simulink model "FOC_2020b"  (R2021a)
settings: Solver=ode23t  StartTime=0.0  StopTime=0.1  RelTol=1e-3  AbsTol=1e-3  EnableMultiTasking=on
values from neighbouring files (symbols this model uses):
  f_c = 10000    [FOC_params.m]
  Kpd = Ld*2*pi*BW    (= 0.0753982236862)    [FOC_params.m]
  Kpn = Kpq/(Lq*d*K)    (= 1.22461076833)    [FOC_params.m]
  Kpq = Lq*2*pi*BW    (= 0.125663706144)    [FOC_params.m]
  Kr = 270    [FOC_params.m]
  Ld = 0.00003    (= 3e-05)    [FOC_params.m]
  Lq = 0.00005    (= 5e-05)    [FOC_params.m]
  np = 5    [FOC_params.m]
  PERIOD = 3750    [FOC_params.m]
  psiPM = 0.007    [FOC_params.m]
  R = 0.023    [FOC_params.m]
  T_dead = 2.0e-6    (= 2e-06)    [FOC_params.m]
  Tnd = Ld/R    (= 0.00130434782609)    [FOC_params.m]
  Tnn = d^2*Lq/Kpq    (= 0.039788735773)    [FOC_params.m]
  Tnq = Lq/R    (= 0.00217391304348)    [FOC_params.m]
  u_dc = 12    [FOC_params.m]
libraries: nesl_utility x23, ee_lib x22, fl_lib x22, pid_lib x3, simulink x3, cstblocks x2, spsAlphaBetaZerotodq0Lib x1, spsabctoAlphaBetaZeroLib x1, spsdq0toAlphaBetaZeroLib x1, spsTriangleGeneratorLib x1
(part 1 of 2)
settings Model: Creator=Michael Hoerner  LastModifiedBy=wilflingti
settings SolverCC: AutoScaleAbsTol=off  AlgebraicLoopSolver=TrustRegion  DecoupledContinuousIntegration=on  MinimalZcImpactIntegration=on
settings DataIOCC: LimitDataPoints=on  MaxDataPoints=10000  ReturnWorkspaceOutputs=off
settings OptimizationCC: StrengthReduction=on  PassReuseOutputArgsAs=Individual arguments  OptimizeBlockOrder=speed  OptimizationPriority=Speed  OptimizationCustomize=off  MultiThreadedLoops=on  EfficientTunableParamExpr=on
settings DebuggingCC: ParameterTunabilityLossMsg=error  AllowSymbolicDim=off  SFUnexpectedBacktrackingDiag=warning  SFNoUnconditionalDefaultTransitionDiag=warning  SFExecutionAtInitializationDiag=none  SFMachineParentedDataDiag=warning  ArithmeticOperatorsInVariantConditions=warning
settings HardwareCC: ProdBitPerChar=16  ProdBitPerInt=16  ProdBitPerPointer=32  ProdBitPerSizeT=32  ProdBitPerPtrDiffT=32  ProdLargestAtomicInteger=Integer  ProdLargestAtomicFloat=None  ProdWordSize=16  ProdHWDeviceType=Texas Instruments->C2000
settings SFSimCC: SimUseLocalCustomCode=off  MATLABDynamicMemAlloc=off  CustomCodeUndefinedFunction=UseInterfaceOnly
settings RTWCC: SystemTargetFile=ert.tlc  TemplateMakefile=ert_default_tmf  GenerateReport=on  RTWUseLocalCustomCode=off  IncludeHyperlinkInReport=on  LaunchReport=on  GenerateTraceInfo=on  GenerateTraceReport=on  GenerateTraceReportSl=on  GenerateTraceReportSf=on  GenerateTraceReportEml=on
settings CodeAppCC: ForceParamTrailComments=on  IgnoreCustomStorageClasses=off  OperatorAnnotations=on  SimulinkDataObjDesc=on  SFDataObjDesc=on  InsertBlockDesc=on
settings ERTTargetCC: CodeReplacementLibrary=TI C28x with C99 extensions  GenerateSampleERTMain=on  CodeInterfacePackaging=Reusable function  MultiInstanceErrorCode=Warning  ERTCustomFileTemplate=example_file_process.tlc  ERTFilePackagingFormat=Compact
settings ConfigComp: CovMetricSettings=dw  CovSaveCumulativeToWorkspaceVar=on  CovSaveSingleToWorkspaceVar=on  CovExternalEMLEnable=off  CovSFcnEnable=off
settings SimscapeCC: SimscapeLogDataHistory=10000

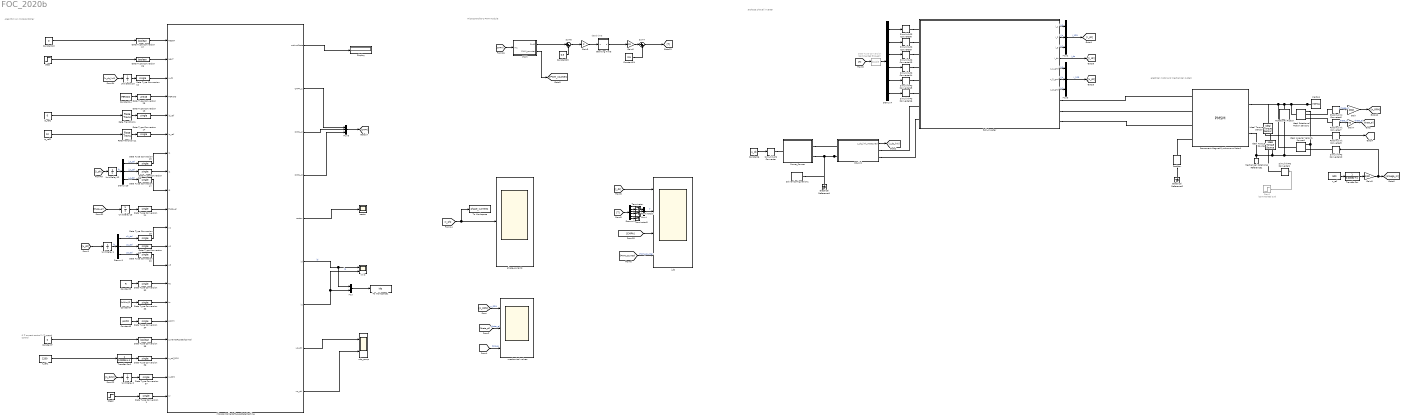
== system FOC_2020b ==
  note: electrical motor and mechanical system
  note: 3-phase 2-level inverter
  note: dead time
  note: Microcontroller's PWM module
  note: Algorithm on microcontroller
  note: 0 = current control
      | 1 = speed control
  3ph_Inverter : Subsystem
  Blanking Time : Subsystem  mask(Blanking Time){tb=T_dead}
      mask prompts: tb "Delay time:"
      mask help:
      | This block generates a blanking time for two-level inverter bridges so that the turn-on of one switch is delayed with respect to the turn-off of the other switch in the inverter leg.
      |
      | The input s is a switching function generated by a 2-level modulator. The values of the output s' are either 1, 0 or -1. If the input is a vector, the output is also a vector of the same width.
      mask Help: eval('plecs(''help'', ''blankingtime.html'')')
  Constant10 : Constant  Value=0
  Constant14 : Constant  Value=PERIOD
  Constant23 : Constant  Value=0.5
  Constant24 : Constant  Value=0.5
  Constant3 : Constant  Value=R
  Constant4 : Constant  Value=(Ld+Lq)/2
  Constant5 : Constant  Value=psiPM
  Constant6 : Constant  Value=u_dc
  Constant7 : Constant  Value=0
  DC_link : Subsystem
  Data Type Conversion : DataTypeConversion  Commented=through  OutDataTypeStr=double
  Data Type Conversion{1,12..21,32..34,36..37} (16 alike) : DataTypeConversion  OutDataTypeStr=single
  Data Type Conversion25 : DataTypeConversion  OutDataTypeStr=uint16
  Data Type Conversion26 : DataTypeConversion  OutDataTypeStr=boolean
  Data Type Conversion27 : DataTypeConversion  OutDataTypeStr=boolean
  Data Type Conversion35 : DataTypeConversion  OutDataTypeStr=boolean
  Demux1 : Demux  Outputs=3
  Demux10 : Demux  Outputs=3
  Demux3 : Demux  Outputs=6
  Demux4 : Demux  Outputs=6
  Display : Display
  Electrical Reference1 : fl_lib/Electrical/Electrical Elements/Electrical Reference
  Electrical Reference2 : fl_lib/Electrical/Electrical Elements/Electrical Reference
  Gain : Gain  Gain=30/pi
  Gain5 : Gain  Gain=2
  Gain6 : Gain  Gain=0.5
  Gain7 : Gain  Gain=np
  Gain8 : Gain  Gain=pi/30
  Ideal Angular Velocity Source1 : fl_lib/Mechanical/Mechanical Sources/Ideal Angular Velocity Source
  Ideal Rotational Motion Sensor1 : fl_lib/Mechanical/Mechanical Sensors/Ideal Rotational Motion Sensor  wrap_angle=simscape.enum.onoff.off  offset=0 deg
  Ideal Torque Sensor : fl_lib/Mechanical/Mechanical Sensors/Ideal Torque Sensor
  Ideal Torque Source : fl_lib/Mechanical/Mechanical Sources/Ideal Torque Source
  Inertia1 : fl_lib/Mechanical/Rotational Elements/Inertia  inertia=J kg*m^2  num_ports=foundation.enum.numPorts2.one  w_specify=off  w_priority=High  w=0 rad/s  w_nominal_specify=off  w_nominal_unit=rad/s  w_nominal_value=1  t_specify=off  t_priority=None  t=0 N*m  t_nominal_specify=off  t_nominal_unit=N*m  t_nominal_value=1
  Mechanical Rotational Reference1 : fl_lib/Mechanical/Rotational Elements/Mechanical Rotational Reference
  MicrocontrollerSoftwareStateMachine : Stateflow chart  TreatAsAtomicUnit=on
  Mux : Mux  Inputs=2
  Mux{2..4,6} (4 alike) : Mux  Inputs=3
  PS-Simulink Converter6 : nesl_utility/PS-Simulink Converter  PhysicalDomain=network_engine_domain  SubClassName=ps_output  LeftPortType=input  RightPortType=output  PseudoPeriodic=off  Frequencies=[]  Unit=1  AffineConversion=off
      settings: SourceProductBaseCode=PW,SS
  PS-Simulink Converter7 : nesl_utility/PS-Simulink Converter  PhysicalDomain=network_engine_domain  SubClassName=ps_output  LeftPortType=input  RightPortType=output  PseudoPeriodic=off  Frequencies=[]  Unit=1  AffineConversion=off
      settings: SourceProductBaseCode=PW,SS
  PS-Simulink Converter8 : nesl_utility/PS-Simulink Converter  PhysicalDomain=network_engine_domain  SubClassName=ps_output  LeftPortType=input  RightPortType=output  PseudoPeriodic=off  Frequencies=[]  Unit=1  AffineConversion=off
      settings: SourceProductBaseCode=PW,SS
  PWM : Subsystem
  Permanent Magnet Synchronous Motor1 : ee_lib/Electromechanical/Permanent Magnet/PMSM  winding_type=ee.enum.statorconnection.wye  machine_param=ee.enum.pmsm.parameterization.constant  nPolePairs=np  pmflux_param=1  pm_flux_linkage=psiPM Wb  torque_constant=0.18 N*m/A  back_emf_constant=0.18 V/(rad/s)  stator_param=1  Ld=Ld H  Lq=Lq H  idVec=[-200, 0, 200] A  iqVec=[-200, 0, 200] A  LdMatrix=0.0002 * ones(3, 3) H  LqMatrix=0.0002 * ones(3, 3) H  PmMatrix=0.1 * ones(3, 3) Wb  ktMatrix=0.18 * ones(3, 3) N*m/A  keMatrix=0.18 * ones(3, 3) V/(rad/s)  L0=0.00016 H  Ls=0.0002 H  Lm=-0.00002 H  Ms=0.00002 H  Rs=R Ohm  zero_sequence=ee.enum.park.zerosequence.include  J=0.0 kg*m^2  lam=0 N*m/(rad/s)  axes_param=2  i_d_specify=off  i_d_priority=None  i_d=0 A  i_d_nominal_specify=off  i_d_nominal_unit=A  i_d_nominal_value=1  i_q_specify=off  i_q_priority=None  i_q=0 A  i_q_nominal_specify=off  i_q_nominal_unit=A  i_q_nominal_value=1  torque_specify=off  torque_priority=None  torque=0 N*m  torque_nominal_specify=off  torque_nominal_unit=N*m  torque_nominal_value=1  angular_velocity_specify=off  angular_velocity_priority=High  angular_velocity=0 deg/s  angular_velocity_nominal_specify=off  angular_velocity_nominal_unit=rpm  angular_velocity_nominal_value=1  angular_position_specify=off  angular_position_priority=High  angular_position=0 deg  angular_position_nominal_specify=off  angular_position_nominal_unit=deg  angular_position_nominal_value=1  loss_param=ee.enum.ironloss.none  losses_oc=[0, 0, 0] W  losses_sc=[0, 0, 0] W  f_losses=60 Hz  Isc_losses=95 A  Tmeas=298.15 K  alpha=3.93e-3 1/K  alpha_flux=-0.001 1/K  stator_thermal_mass=100 J/K  rotor_thermal_mass=200 J/K  Rm_percent_rotor=90  Rd_percent_rotor=30  temperatureA_specify=off  temperatureA_priority=High  temperatureA=25 degC  temperatureA_nominal_specify=off  temperatureA_nominal_unit=degC  temperatureA_nominal_value=1  temperatureB_specify=off  temperatureB_priority=High  temperatureB=25 degC  temperatureB_nominal_specify=off  temperatureB_nominal_unit=degC  temperatureB_nominal_value=1  temperatureC_specify=off  temperatureC_priority=High  temperatureC=25 degC  temperatureC_nominal_specify=off  temperatureC_nominal_unit=degC  temperatureC_nominal_value=1  temperatureR_specify=off  temperatureR_priority=High  temperatureR=25 degC  temperatureR_nominal_specify=off  temperatureR_nominal_unit=degC  temperatureR_nominal_value=1
      settings: InternalSimscapePortConfiguration="{\"Bottom\":[],\"Left\":[{\"id\":\"a\",\"label\":\"a\",\"type\":\"foundation.electrical.electrical\"},{\"id\":\"b\",\"label\":\"b\",\"type\":\"foundation.electrical.electrical\"},{\"id\":\"c\",\"label\":\"c\",\"type\":\"foundation.electrical.electrical\"},{\"id\":\"n\",\"label\":\"n\",\"type\":\"foundation.electrical.electrical\"}],\"Right\":[{\"id\":\"R\",\"label\":\"R\",\"type\":\"foundation.mechanical.rotational.rotational\"},{\"id\":\"C\",\"label\":\"C\",\"type\":\"foundation.mechanical.rotational.rotational\"}],\"Top\":[]}"
  Power_Source : Subsystem
  Rate Transition1 : RateTransition  OutPortSampleTime=1/f_c
  Rate Transition11 : RateTransition  OutPortSampleTime=1/f_c
  Resistor : fl_lib/Electrical/Electrical Elements/Resistor  R=2e6 Ohm  i_specify=off  i_priority=None  i=0 A  i_nominal_specify=off  i_nominal_unit=A  i_nominal_value=1  v_specify=off  v_priority=None  v=0 V  v_nominal_specify=off  v_nominal_unit=V  v_nominal_value=1
  Rotational Friction : fl_lib/Mechanical/Rotational Elements/Rotational Friction  brkwy_trq=0.0622476 N*m  brkwy_vel=0.1 rad/s  Col_trq=0.03460117 N*m  visc_coef=0.00026373 N*m/(rad/s)  w_specify=off  w_priority=None  w=0 rad/s  w_nominal_specify=off  w_nominal_unit=rad/s  w_nominal_value=1  t_specify=off  t_priority=None  t=0 N*m  t_nominal_specify=off  t_nominal_unit=N*m  t_nominal_value=1
  Simulink-PS Converter{,8..9,13..16} (7 alike) : nesl_utility/Simulink-PS Converter  PhysicalDomain=network_engine_domain  SubClassName=ps_input  LeftPortType=input  RightPortType=output  PseudoPeriodic=off  Frequencies=[]  NoiseDistribution=none  NoiseParameters=[]  Unit=1  AffineConversion=off  FilteringAndDerivatives=provide  SimscapeFilterOrder=1  InputFilterTimeConstant=0.001  UdotUserProvided=0
      settings: SourceProductBaseCode=PW,SS
  Simulink-PS Converter1 : nesl_utility/Simulink-PS Converter  PhysicalDomain=network_engine_domain  SubClassName=ps_input  LeftPortType=input  RightPortType=output  PseudoPeriodic=off  Frequencies=[]  NoiseDistribution=none  NoiseParameters=[]  Unit=1  AffineConversion=off  FilteringAndDerivatives=filter  SimscapeFilterOrder=1  InputFilterTimeConstant=0.001  UdotUserProvided=0
      settings: SourceProductBaseCode=PW,SS
  Simulink-PS Converter10 : nesl_utility/Simulink-PS Converter  PhysicalDomain=network_engine_domain  SubClassName=ps_input  LeftPortType=input  RightPortType=output  PseudoPeriodic=off  Frequencies=[]  NoiseDistribution=none  NoiseParameters=[]  Unit=1  AffineConversion=off  FilteringAndDerivatives=filter  SimscapeFilterOrder=1  InputFilterTimeConstant=0.001  UdotUserProvided=0
      settings: SourceProductBaseCode=PW,SS
  Solver Configuration1 : nesl_utility/Solver Configuration  PhysicalDomain=network_engine_domain  SubClassName=solver  LeftPortType=input  RightPortType=generic  Tones=[]  Harmonics=[]  SimulateNoise=off  Profile=off  UseLocalSampling=off  EnableSwitchedLinearOptims=on  FrequencyDomain=off  UseCCode=off  RelTol=0.001  AbsTol=1e-06  MinStep=1e-09  ToWorkspace=off  RevertToSquareIcSolve=off  NumHomotopyIterations=100  PhasorMode=off  PhasorModeNumHarmonics=1  DoDC=off  ResidualTolerance=1e-09  UseLocalSolver=off  LocalSolverChoice=NE_BACKWARD_EULER_ADVANCER  LocalSolverSampleTime=1e-6  DoFixedCost=off  MaxNonlinIter=3  MaxModeIter=2  ComputeImpulses=off  ImpulseIterations=2  LinearAlgebra=Sparse  EquationFormulation=NE_TIME_EF  DelaysMemoryBudget=1024  AutomaticFiltering=on  FilteringTimeConstant=0.001  PartitionStorageMethod=AS_NEEDED  PartitionMemoryBudget=1024  PartitionMethod=FAST
      settings: SourceProductBaseCode=PW,SS
  Step : Step  Time=2/f_c  Before=1  After=0  SampleTime=0
  Step1 : Step  Commented=on  Time=0.08  After=-0.5  SampleTime=0
  Step2 : Step  Time=0.04  After=Kr  SampleTime=0
  Sum6 : Sum  Inputs=|+-
  Sum7 : Sum  Inputs=|++
  Terminator : Terminator
  Terminator1 : Terminator
  Terminator3 : Terminator
  To Workspace : ToWorkspace  VariableName=phase_currents  SaveFormat=Timeseries  SampleTime=1/1000
  To Workspace1 : ToWorkspace  VariableName=idq  SaveFormat=Timeseries  SampleTime=1/1000
  Transfer Fcn : TransferFcn  Denominator=[0.0005 1]
  Transfer Fcn1 : TransferFcn  Denominator=[0.0005 1]
  Unit Delay{1..2,10,12..13} (5 alike) : UnitDelay  SampleTime=1/f_c  HasFrameUpgradeWarning=on
  i_dc : Scope  NumInputPorts=4
  id,iq : Scope  NumInputPorts=2
  id_ref2 : Constant  Value=0
  iq_ref2 : Constant  Value=10
  mechanical values : Scope  NumInputPorts=3
  n_ref : Constant  Value=500
  n_ref1 : Constant  Value=1200
  phase_currents : Scope
  "sector " : Scope
  udq_comp : Scope  NumInputPorts=2
  wires:
  DC_link/1(u_dc_link_measured) -> [u_dc_link]
  Constant6/1 -> Simulink-PS Converter/1
  3ph_Inverter/3(i_3) -> Mux2/3  "i_c"
  3ph_Inverter/2(i_2) -> Mux2/2  "i_b"
  Mux2/1 -> [i_ph]  "i_123"
  PS-Simulink Converter7/1 -> Gain7/1  "theta_m"
  Gain7/1 -> [theta_el]  "theta_el"
  Gain8/1 -> Simulink-PS Converter10/1, [omega_m]
  PS-Simulink Converter6/1 -> Gain/1  "omega_m"
  PS-Simulink Converter8/1 -> [torque]
  [T] -> Demux3/1
  Demux3/1 -> Mux4/1
  Demux3/3 -> Mux4/2
  Demux3/5 -> Mux4/3
  Demux3/2 -> Terminator/1
  Demux3/4 -> Terminator1/1
  [PWM_counter] -> i_dc/4  "PWM_counter"
  3ph_Inverter/1(i_1) -> Mux2/1  "i_a"
  3ph_Inverter/4(i_dc) -> [i_dc]  "i_dc"
  [i_dc] -> i_dc/1
  Demux3/6 -> Terminator3/1
  [T] -> Data Type Conversion/1
  [i_ph] -> To Workspace/1, phase_currents/1
  Mux4/1 -> i_dc/2  "T"
  n_ref/1 -> Transfer Fcn/1
  Data Type Conversion12/1 -> MicrocontrollerSoftwareStateMachine/3(u_dc)
  Data Type Conversion13/1 -> MicrocontrollerSoftwareStateMachine/5(id_ref)
  Data Type Conversion14/1 -> MicrocontrollerSoftwareStateMachine/6(iq_ref)
  Data Type Conversion15/1 -> MicrocontrollerSoftwareStateMachine/7(i1)
  Data Type Conversion16/1 -> MicrocontrollerSoftwareStateMachine/8(i2)
  Data Type Conversion17/1 -> MicrocontrollerSoftwareStateMachine/9(i3)
  Data Type Conversion21/1 -> MicrocontrollerSoftwareStateMachine/10(theta_el)
  Data Type Conversion25/1 -> MicrocontrollerSoftwareStateMachine/4(PERIOD)
  Data Type Conversion26/1 -> MicrocontrollerSoftwareStateMachine/2(NEXT)
  Data Type Conversion27/1 -> MicrocontrollerSoftwareStateMachine/1(RESET)
  Constant10/1 -> Data Type Conversion27/1
  Step/1 -> Data Type Conversion26/1
  Unit Delay10/1 -> Data Type Conversion12/1
  [u_dc_link] -> Unit Delay10/1
  Constant14/1 -> Data Type Conversion25/1
  Rate Transition11/1 -> Data Type Conversion14/1
  id_ref2/1 -> Rate Transition1/1
  iq_ref2/1 -> Rate Transition11/1
  Rate Transition1/1 -> Data Type Conversion13/1
  Demux10/3 -> Data Type Conversion17/1  "i_c_ctrl"
  Unit Delay12/1 -> Demux10/1  "fc"
  Demux10/1 -> Data Type Conversion15/1  "i_a_ctrl"
  Demux10/2 -> Data Type Conversion16/1  "i_b_ctrl"
  [i_ph] -> Unit Delay12/1
  [theta_el] -> Unit Delay13/1
  Unit Delay13/1 -> Data Type Conversion21/1
  MicrocontrollerSoftwareStateMachine/3(CMPA_2) -> Mux6/2
  MicrocontrollerSoftwareStateMachine/2(CMPA_1) -> Mux6/1
  MicrocontrollerSoftwareStateMachine/4(CMPA_3) -> Mux6/3
  MicrocontrollerSoftwareStateMachine/5(sector) -> "sector "/1
  Transfer Fcn/1 -> Gain8/1
  [CMPA] -> i_dc/3
  Mux6/1 -> [CMPA]
  Demux1/2 -> Data Type Conversion19/1  "u2_ctrl"
  Unit Delay1/1 -> Demux1/1  "fc"
  Demux1/1 -> Data Type Conversion18/1  "u1_ctrl"
  [u_ph] -> Unit Delay1/1
  Demux1/3 -> Data Type Conversion20/1  "u3_ctrl"
  Data Type Conversion19/1 -> MicrocontrollerSoftwareStateMachine/12(u2)
  Data Type Conversion18/1 -> MicrocontrollerSoftwareStateMachine/11(u1)
  Data Type Conversion20/1 -> MicrocontrollerSoftwareStateMachine/13(u3)
  Data Type Conversion32/1 -> MicrocontrollerSoftwareStateMachine/14(Rs)
  Data Type Conversion33/1 -> MicrocontrollerSoftwareStateMachine/15(Ls)
  Data Type Conversion34/1 -> MicrocontrollerSoftwareStateMachine/16(psiPM)
  Constant3/1 -> Data Type Conversion32/1
  Constant4/1 -> Data Type Conversion33/1
  Constant5/1 -> Data Type Conversion34/1
  3ph_Inverter/5(u_1_gnd) -> Mux3/1  "i_a"
  Mux3/1 -> [u_ph]  "i_123"
  3ph_Inverter/6(u_2_gnd) -> Mux3/2  "i_b"
  3ph_Inverter/7(u_3_gnd) -> Mux3/3  "i_c"
  Data Type Conversion35/1 -> MicrocontrollerSoftwareStateMachine/17(currentORspeedControl)
  Data Type Conversion36/1 -> MicrocontrollerSoftwareStateMachine/18(n_ref_RPM)
  Data Type Conversion37/1 -> MicrocontrollerSoftwareStateMachine/19(n_RPM)
  Constant7/1 -> Data Type Conversion35/1
  Gain/1 -> [n_RPM]
  Unit Delay2/1 -> Data Type Conversion37/1
  [n_RPM] -> Unit Delay2/1
  Transfer Fcn1/1 -> Data Type Conversion36/1
  Step1/1 -> Simulink-PS Converter1/1
  MicrocontrollerSoftwareStateMachine/6(id) -> Mux/1, id,iq/1  "id"
  MicrocontrollerSoftwareStateMachine/7(iq) -> Mux/2, id,iq/2  "iq"
  Data Type Conversion/1 -> Demux4/1
  PWM/2(PWM_counter) -> [PWM_counter]
  Demux4/1 -> Simulink-PS Converter8/1
  Demux4/2 -> Simulink-PS Converter9/1
  Demux4/3 -> Simulink-PS Converter13/1
  Demux4/4 -> Simulink-PS Converter14/1
  Demux4/5 -> Simulink-PS Converter15/1
  Demux4/6 -> Simulink-PS Converter16/1
  Gain5/1 -> Blanking Time/1(s)
  Constant23/1 -> Sum6/2
  Gain6/1 -> Sum7/1
  Blanking Time/1(s') -> Gain6/1
  Constant24/1 -> Sum7/2
  Sum6/1 -> Gain5/1
  Sum7/1 -> [T]
  PWM/1(Out1) -> Sum6/1
  MicrocontrollerSoftwareStateMachine/8(ud_ctrl) -> udq_comp/1
  MicrocontrollerSoftwareStateMachine/9(uq_ctrl) -> udq_comp/2
  n_ref1/1 -> Transfer Fcn1/1
  [CMPA] -> PWM/1(In1)
  MicrocontrollerSoftwareStateMachine/1(activeState) -> Display/1
  [torque] -> mechanical values/3  "torque"
  [n_RPM] -> mechanical values/1  "n_RPM"
  [theta_el] -> mechanical values/2  "theta_el"
  Data Type Conversion1/1 -> MicrocontrollerSoftwareStateMachine/20(Kr)
  Step2/1 -> Data Type Conversion1/1
  Mux/1 -> To Workspace1/1
  connections:
  DC_link/LConn2 -- Power_Source/RConn2 -- Solver Configuration1/RConn1 -- Electrical Reference1/LConn1
  Inertia1/LConn1 -- Ideal Angular Velocity Source1/LConn1 -- Permanent Magnet Synchronous Motor1/RConn1 -- Ideal Torque Sensor/LConn1 -- Rotational Friction/LConn1 -- Ideal Rotational Motion Sensor1/LConn1
  Ideal Rotational Motion Sensor1/RConn1 -- Ideal Angular Velocity Source1/RConn2 -- Rotational Friction/RConn1 -- Permanent Magnet Synchronous Motor1/RConn2 -- Mechanical Rotational Reference1/LConn1 -- Ideal Torque Source/RConn2
  Simulink-PS Converter14/RConn1 -- 3ph_Inverter/LConn4
  Simulink-PS Converter15/RConn1 -- 3ph_Inverter/LConn5
  Simulink-PS Converter16/RConn1 -- 3ph_Inverter/LConn6
  Power_Source/RConn1 -- DC_link/LConn1
  PS-Simulink Converter6/LConn1 -- Ideal Rotational Motion Sensor1/RConn2
  Simulink-PS Converter/RConn1 -- Power_Source/LConn1
  Simulink-PS Converter8/RConn1 -- 3ph_Inverter/LConn1
  Simulink-PS Converter9/RConn1 -- 3ph_Inverter/LConn2
  DC_link/RConn1 -- 3ph_Inverter/LConn7
  Simulink-PS Converter13/RConn1 -- 3ph_Inverter/LConn3
  DC_link/RConn2 -- 3ph_Inverter/LConn8
  PS-Simulink Converter7/LConn1 -- Ideal Rotational Motion Sensor1/RConn3
  3ph_Inverter/RConn1 -- Permanent Magnet Synchronous Motor1/LConn1
  3ph_Inverter/RConn2 -- Permanent Magnet Synchronous Motor1/LConn2
  3ph_Inverter/RConn3 -- Permanent Magnet Synchronous Motor1/LConn3
  Resistor/LConn1 -- Permanent Magnet Synchronous Motor1/LConn4
  Simulink-PS Converter10/RConn1 -- Ideal Angular Velocity Source1/RConn1
  PS-Simulink Converter8/LConn1 -- Ideal Torque Sensor/RConn2
  Resistor/RConn1 -- Electrical Reference2/LConn1
  Simulink-PS Converter1/RConn1 -- Ideal Torque Source/RConn1
  Ideal Torque Source/LConn1 -- Ideal Torque Sensor/RConn1

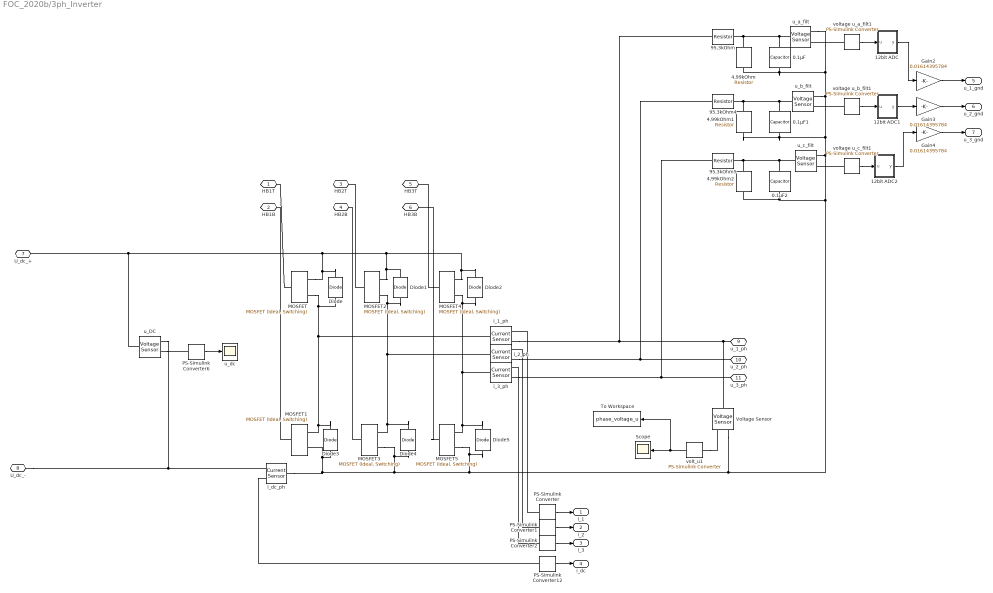
== system FOC_2020b/3ph_Inverter ==
  0.1µF : ee_lib/Passive/Capacitor  cap_option=0  c=0.1 uF  Cvec=[ 1e-5 1e-6 ] F  Vvec=[ 0 10 ] V  CV_table_symmetry=1  f_vec=[1, 10] kHz  DFext_vec=[.8, 1.2]  C_tol=5  enable_C_tol=0  tol_distribution=1  nSigma=4  r=1e-6 Ohm  g=0 1/Ohm  averaging_period=0 s  enable_operating_limits=0  operating_limit_action=2  max_working_voltage_range=[ -25 25 ] V  power_rating=1 W  enable_faults=0  fault_action=1  Cscale_faulted=100  R_faulted=0.001 Ohm  G_faulted=0 1/Ohm  tau_fault=0.001 s  enable_temporal_fault=0  t_fault=1 s  enable_behavioral_fault=0  max_permissible_voltage_range=[ -100 100 ] V  t_fail_on_voltage=1 s  i_specify=off  i_priority=None  i=0 A  i_nominal_specify=off  i_nominal_unit=A  i_nominal_value=1  v_specify=off  v_priority=None  v=0 V  v_nominal_specify=off  v_nominal_unit=V  v_nominal_value=1  vc_specify=on  vc_priority=High  vc=0 V  vc_nominal_specify=off  vc_nominal_unit=V  vc_nominal_value=1
  0.1µF1 : ee_lib/Passive/Capacitor  cap_option=0  c=0.1 uF  Cvec=[ 1e-5 1e-6 ] F  Vvec=[ 0 10 ] V  CV_table_symmetry=1  f_vec=[1, 10] kHz  DFext_vec=[.8, 1.2]  C_tol=5  enable_C_tol=0  tol_distribution=1  nSigma=4  r=1e-6 Ohm  g=0 1/Ohm  averaging_period=0 s  enable_operating_limits=0  operating_limit_action=2  max_working_voltage_range=[ -25 25 ] V  power_rating=1 W  enable_faults=0  fault_action=1  Cscale_faulted=100  R_faulted=0.001 Ohm  G_faulted=0 1/Ohm  tau_fault=0.001 s  enable_temporal_fault=0  t_fault=1 s  enable_behavioral_fault=0  max_permissible_voltage_range=[ -100 100 ] V  t_fail_on_voltage=1 s  i_specify=off  i_priority=None  i=0 A  i_nominal_specify=off  i_nominal_unit=A  i_nominal_value=1  v_specify=off  v_priority=None  v=0 V  v_nominal_specify=off  v_nominal_unit=V  v_nominal_value=1  vc_specify=on  vc_priority=High  vc=0 V  vc_nominal_specify=off  vc_nominal_unit=V  vc_nominal_value=1
  0.1µF2 : ee_lib/Passive/Capacitor  cap_option=0  c=0.1 uF  Cvec=[ 1e-5 1e-6 ] F  Vvec=[ 0 10 ] V  CV_table_symmetry=1  f_vec=[1, 10] kHz  DFext_vec=[.8, 1.2]  C_tol=5  enable_C_tol=0  tol_distribution=1  nSigma=4  r=1e-6 Ohm  g=0 1/Ohm  averaging_period=0 s  enable_operating_limits=0  operating_limit_action=2  max_working_voltage_range=[ -25 25 ] V  power_rating=1 W  enable_faults=0  fault_action=1  Cscale_faulted=100  R_faulted=0.001 Ohm  G_faulted=0 1/Ohm  tau_fault=0.001 s  enable_temporal_fault=0  t_fault=1 s  enable_behavioral_fault=0  max_permissible_voltage_range=[ -100 100 ] V  t_fail_on_voltage=1 s  i_specify=off  i_priority=None  i=0 A  i_nominal_specify=off  i_nominal_unit=A  i_nominal_value=1  v_specify=off  v_priority=None  v=0 V  v_nominal_specify=off  v_nominal_unit=V  v_nominal_value=1  vc_specify=on  vc_priority=High  vc=0 V  vc_nominal_specify=off  vc_nominal_unit=V  vc_nominal_value=1
  12bit ADC : MATLAB Function  TreatAsAtomicUnit=on
  12bit ADC1 : MATLAB Function  TreatAsAtomicUnit=on
  12bit ADC2 : MATLAB Function  TreatAsAtomicUnit=on
  4,99kOhm : ee_lib/Passive/Resistor  R=4990 Ohm  R_tol=5  enable_R_tol=0  tol_distribution=1  nSigma=4  enable_operating_limits=0  operating_limit_action=2  max_working_voltage=100 V  power_rating=1 W  enable_faults=0  fault_action=1  R_faulted=Inf Ohm  enable_temporal_fault=0  t_fault=1 s  enable_behavioral_fault=0  max_permissible_current=1 A  t_fail_on_current=1 s  noise_mode=0  sample_time=0.001 s  repeatability=1  auto_seed=785646024  user_seed=0  Tdevice=25 degC  alpha=3.93e-3 1/K  Tmeas=25 degC  thermal_mass=100 J/K  power_derating_T1=70 degC  power_derating_T2=155 degC  operating_temperature_range_vec=[-50, 150] degC  temperature_specify=off  temperature_priority=High  temperature=298.15 K  temperature_nominal_specify=off  temperature_nominal_unit=K  temperature_nominal_value=1
  4,99kOhm1 : ee_lib/Passive/Resistor  R=4990 Ohm  R_tol=5  enable_R_tol=0  tol_distribution=1  nSigma=4  enable_operating_limits=0  operating_limit_action=2  max_working_voltage=100 V  power_rating=1 W  enable_faults=0  fault_action=1  R_faulted=Inf Ohm  enable_temporal_fault=0  t_fault=1 s  enable_behavioral_fault=0  max_permissible_current=1 A  t_fail_on_current=1 s  noise_mode=0  sample_time=0.001 s  repeatability=1  auto_seed=1030500139  user_seed=0  Tdevice=25 degC  alpha=3.93e-3 1/K  Tmeas=25 degC  thermal_mass=100 J/K  power_derating_T1=70 degC  power_derating_T2=155 degC  operating_temperature_range_vec=[-50, 150] degC  temperature_specify=off  temperature_priority=High  temperature=298.15 K  temperature_nominal_specify=off  temperature_nominal_unit=K  temperature_nominal_value=1
  4,99kOhm2 : ee_lib/Passive/Resistor  R=4990 Ohm  R_tol=5  enable_R_tol=0  tol_distribution=1  nSigma=4  enable_operating_limits=0  operating_limit_action=2  max_working_voltage=100 V  power_rating=1 W  enable_faults=0  fault_action=1  R_faulted=Inf Ohm  enable_temporal_fault=0  t_fault=1 s  enable_behavioral_fault=0  max_permissible_current=1 A  t_fail_on_current=1 s  noise_mode=0  sample_time=0.001 s  repeatability=1  auto_seed=3807539760  user_seed=0  Tdevice=25 degC  alpha=3.93e-3 1/K  Tmeas=25 degC  thermal_mass=100 J/K  power_derating_T1=70 degC  power_derating_T2=155 degC  operating_temperature_range_vec=[-50, 150] degC  temperature_specify=off  temperature_priority=High  temperature=298.15 K  temperature_nominal_specify=off  temperature_nominal_unit=K  temperature_nominal_value=1
  95,3kOhm : ee_lib/Passive/Resistor  R=95300 Ohm  R_tol=5  enable_R_tol=0  tol_distribution=1  nSigma=4  enable_operating_limits=0  operating_limit_action=2  max_working_voltage=100 V  power_rating=1 W  enable_faults=0  fault_action=1  R_faulted=Inf Ohm  enable_temporal_fault=0  t_fault=1 s  enable_behavioral_fault=0  max_permissible_current=1 A  t_fail_on_current=1 s  noise_mode=0  sample_time=0.001 s  repeatability=1  auto_seed=123154548  user_seed=0  Tdevice=25 degC  alpha=3.93e-3 1/K  Tmeas=25 degC  thermal_mass=100 J/K  power_derating_T1=70 degC  power_derating_T2=155 degC  operating_temperature_range_vec=[-50, 150] degC  temperature_specify=off  temperature_priority=High  temperature=298.15 K  temperature_nominal_specify=off  temperature_nominal_unit=K  temperature_nominal_value=1
  95,3kOhm4 : ee_lib/Passive/Resistor  R=95300 Ohm  R_tol=5  enable_R_tol=0  tol_distribution=1  nSigma=4  enable_operating_limits=0  operating_limit_action=2  max_working_voltage=100 V  power_rating=1 W  enable_faults=0  fault_action=1  R_faulted=Inf Ohm  enable_temporal_fault=0  t_fault=1 s  enable_behavioral_fault=0  max_permissible_current=1 A  t_fail_on_current=1 s  noise_mode=0  sample_time=0.001 s  repeatability=1  auto_seed=2104110442  user_seed=0  Tdevice=25 degC  alpha=3.93e-3 1/K  Tmeas=25 degC  thermal_mass=100 J/K  power_derating_T1=70 degC  power_derating_T2=155 degC  operating_temperature_range_vec=[-50, 150] degC  temperature_specify=off  temperature_priority=High  temperature=298.15 K  temperature_nominal_specify=off  temperature_nominal_unit=K  temperature_nominal_value=1
  95,3kOhm5 : ee_lib/Passive/Resistor  R=95300 Ohm  R_tol=5  enable_R_tol=0  tol_distribution=1  nSigma=4  enable_operating_limits=0  operating_limit_action=2  max_working_voltage=100 V  power_rating=1 W  enable_faults=0  fault_action=1  R_faulted=Inf Ohm  enable_temporal_fault=0  t_fault=1 s  enable_behavioral_fault=0  max_permissible_current=1 A  t_fail_on_current=1 s  noise_mode=0  sample_time=0.001 s  repeatability=1  auto_seed=721241599  user_seed=0  Tdevice=25 degC  alpha=3.93e-3 1/K  Tmeas=25 degC  thermal_mass=100 J/K  power_derating_T1=70 degC  power_derating_T2=155 degC  operating_temperature_range_vec=[-50, 150] degC  temperature_specify=off  temperature_priority=High  temperature=298.15 K  temperature_nominal_specify=off  temperature_nominal_unit=K  temperature_nominal_value=1
  Diode{,1..5} (6 alike) : ee_lib/Semiconductors & Converters/Diode  ModelType=ee.enum.diode.modelType.pwl  IfMat=[.07, .12, .19, 1.75, 4.24, 7.32, 11.2; .16, .3, .72, 2.14, 4.02, 6.35, 9.12] A  TjVec=[25, 125] degC  VfVec=[.5, .7, .9, 1.3, 1.7, 2.1, 2.5] V  Vf=0.1 V  Ron=0.001 Ohm  Goff=1e-5 1/Ohm  prmExp=ee.enum.diode.expParam.useTwo  I12=[.0137, .545] A  V12=[.6, .7] V  IS=1e-12 A  ec=1  I1=0.0137 A  V1=0.6 V  RS=0 Ohm  Tmeas=25 degC  N_series=1  N_parallel=1  Rz=0.3 Ohm  BV=inf V  C_param=ee.enum.diode.capParam.fixed  CJ=0 pF  CJ0=5 pF  VJ=1 V  Mgrad=0.5  Vvec=[.1, 10, 100] V  Cvec=[3.5, 1, .4] pF  FC=0.5  Q_param=ee.enum.diode.recoveryParam.off  iRM=-7.15 A  iF=4 A  didt=-750 A/us  trr_factor=3  trr=115 ns  Qrr=150 s*nA  TT=50 ns  tau=100 ns  T_param=ee.enum.diode.temperatureParam.off  IS_T2=1.25e-7 A  I1_T2=0.245 A  V1_T2=0.5 V  Tmeas2=125 degC  EG_param=ee.enum.diode.egapParam.material_si  EG=1.11 eV  XTI_param=ee.enum.diode.xtiParam.pn  XTI=3  dBVdT=0 V/K  enable_faults=ee.enum.faults.faultEnable.no  fault_action=ee.enum.faults.faultAction.none  fault_types=ee.enum.diode.faults.open  tau_fault=1e-3 s  IfMat_faulted=[.07, .12, .19, 1.75, 4.24, 7.32, 11.2; .16, .3, .72, 2.14, 4.02, 6.35, 9.12] A  VfVec_faulted=[.5, .7, .9, 1.3, 1.7, 2.1, 2.5] V  Ropen_faulted=1000 Ohm  Gshort_faulted=1000 1/Ohm  Vf_faulted=0.6 V  Ron_faulted=0.3 Ohm  Goff_faulted=1e-8 S  I12_faulted=[.0137, .545] A  V12_faulted=[.6, .7] V  IS_faulted=1e-12 A  ec_faulted=1  I1_faulted=0.0137 A  V1_faulted=0.6 V  RS_faulted=0 Ohm  Rz_faulted=0.3 Ohm  BV_faulted=inf V  Cscale_faulted=100  enable_temporal_fault=ee.enum.faults.faultEnable.no  t_fault=inf s  enable_behavioral_fault=ee.enum.faults.faultEnable.no  max_permissible_voltage=inf V  n_fail_on_voltage=1  max_permissible_current=inf A  t_fail_on_current=1 s  max_permissible_dVdt=inf V/s  Tdevice=25 degC  i_specify=off  i_priority=None  i=0 A  i_nominal_specify=off  i_nominal_unit=A  i_nominal_value=1  v_specify=off  v_priority=None  v=0 V  v_nominal_specify=off  v_nominal_unit=V  v_nominal_value=1  i_diode_specify=off  i_diode_priority=None  i_diode=0 A  i_diode_nominal_specify=off  i_diode_nominal_unit=A  i_diode_nominal_value=1  v_diode_specify=off  v_diode_priority=None  v_diode=0 V  v_diode_nominal_specify=off  v_diode_nominal_unit=V  v_diode_nominal_value=1  i_capacitor_specify=off  i_capacitor_priority=None  i_capacitor=0 A  i_capacitor_nominal_specify=off  i_capacitor_nominal_unit=A  i_capacitor_nominal_value=1  v_capacitor_specify=off  v_capacitor_priority=None  v_capacitor=0 V  v_capacitor_nominal_specify=off  v_capacitor_nominal_unit=V  v_capacitor_nominal_value=1  power_dissipated_specify=off  power_dissipated_priority=None  power_dissipated=0 W  power_dissipated_nominal_specify=off  power_dissipated_nominal_unit=W  power_dissipated_nominal_value=1  max_permissible_temperature=inf K  t_fail_on_temperature=1 s  thermal_network_parameterization=ee.enum.thermalNetworkTopology.cauer  Rth=[0, 10] K/W  Rth_Foster=[4, 6] K/W  thermal_mass_parameterization=ee.enum.thermalNetwork.timeconstant  thermal_mass=[0, 1] J/K  thermal_mass_Foster=[1.5, 3] J/K  thermal_time_constant=[0, 10] s  thermal_time_constant_Foster=[6, 18] s  thermal_mass_initial_temperatures=[25, 25] degC
  Gain2 : Gain  Gain=0.01614395784
  Gain3 : Gain  Gain=0.01614395784
  Gain4 : Gain  Gain=0.01614395784
  MOSFET{,1..5} (6 alike) : ee_lib/Semiconductors & Converters/MOSFET (Ideal, Switching)  Rds=0.040 Ohm  Goff=1e-6 1/Ohm  Vth=0.7 V  diode_param=1  diode_Vf=0.8 V  diode_Ron=0.001 Ohm  diode_Goff=1e-5 1/Ohm  diode_C=5e-8 F  diode_iRM=-235 A  diode_iF=300 A  diode_idot=-50 A/us  diode_trr_param=1  diode_trr_factor=3  diode_trr=15 us  diode_Qrr=1.5e+3 s*uA  thermal_loss_option=ee.enum.converters.thermalLossOption.constantvalues  Von_data=[0, 1.1, 1.3, 1.45, 1.75, 2.25, 2.7; 0, 1, 1.15, 1.35, 1.7, 2.35, 3] V  Eon_data=[0, .29, 1.43, 2.86, 5.71, 13.14, 22.86; 0, .57, 2.63, 5.14, 10.29, 20.57, 30.29] * 1e-3 J  Eoff_data=[0, .21, 1.07, 2.14, 4.29, 9.86, 17.14; 0, .43, 1.97, 3.86, 7.71, 15.43, 22.71] * 1e-3 J  Tj=[298.15, 398.15] K  Iout_data=[0, 10, 50, 100, 200, 400, 600] A  Eon_scalar=22.86e-3 J  Eoff_scalar=17.14e-3 J  Voff=300 V  Iout_scalar=600 A  diodeModelType=ee.enum.converters.diodeModelType.pwl  diode_IfMat=[.07, .12, .19, 1.75, 4.24, 7.32, 11.2; .16, .3, .72, 2.14, 4.02, 6.35, 9.12] A  diode_TjVec=[25, 125] degC  diode_VfVec=[.5, .7, .9, 1.3, 1.7, 2.1, 2.5] V  thermal_network_parameterization=ee.enum.thermalNetworkTopology.external  Rth=[.03, .2] K/W  Rth_Foster=[.03, .2] K/W  thermal_mass_parameterization=ee.enum.thermalNetwork.timeconstant  thermal_mass=[3, 25] J/K  thermal_mass_Foster=[33, 50] J/K  thermal_time_constant=[.1, 5] s  thermal_time_constant_Foster=[1, 10] s  thermal_mass_initial_temperatures=[25, 25] degC  junction_thermal_mass=0.1 J/K  vT_specify=off  vT_priority=None  vT=0 V  vT_nominal_specify=off  vT_nominal_unit=V  vT_nominal_value=1  Qj_specify=off  Qj_priority=None  Qj=0 W  Qj_nominal_specify=off  Qj_nominal_unit=W  Qj_nominal_value=1  junction_temperature_specify=off  junction_temperature_priority=None  junction_temperature=25 degC  junction_temperature_nominal_specify=off  junction_temperature_nominal_unit=degC  junction_temperature_nominal_value=1
  PS-Simulink Converter{,1..2,12} (4 alike) : nesl_utility/PS-Simulink Converter  PhysicalDomain=network_engine_domain  SubClassName=ps_output  LeftPortType=input  RightPortType=output  PseudoPeriodic=off  Frequencies=[]  Unit=A  AffineConversion=off
      settings: SourceProductBaseCode=PW,SS
  PS-Simulink Converter6 : nesl_utility/PS-Simulink Converter  PhysicalDomain=network_engine_domain  SubClassName=ps_output  LeftPortType=input  RightPortType=output  PseudoPeriodic=off  Frequencies=[]  Unit=V  AffineConversion=off
      settings: SourceProductBaseCode=PW,SS
  Scope : Scope
  To Workspace : ToWorkspace  VariableName=phase_voltage_u  SaveFormat=Timeseries  SampleTime=-1
  Voltage Sensor : fl_lib/Electrical/Electrical Sensors/Voltage Sensor
  i_1_ph : fl_lib/Electrical/Electrical Sensors/Current Sensor
  i_2_ph : fl_lib/Electrical/Electrical Sensors/Current Sensor
  i_3_ph : fl_lib/Electrical/Electrical Sensors/Current Sensor
  i_dc_ph : fl_lib/Electrical/Electrical Sensors/Current Sensor
  u_DC : fl_lib/Electrical/Electrical Sensors/Voltage Sensor
      settings: LogSimulationData=on
  u_a_filt : fl_lib/Electrical/Electrical Sensors/Voltage Sensor
      settings: LogSimulationData=on
  u_b_filt : fl_lib/Electrical/Electrical Sensors/Voltage Sensor
      settings: LogSimulationData=on
  u_c_filt : fl_lib/Electrical/Electrical Sensors/Voltage Sensor
      settings: LogSimulationData=on
  u_dc : Scope
  volt_u1 : nesl_utility/PS-Simulink Converter  PhysicalDomain=network_engine_domain  SubClassName=ps_output  LeftPortType=input  RightPortType=output  PseudoPeriodic=off  Frequencies=[]  Unit=V  AffineConversion=off
      settings: SourceProductBaseCode=PW,SS
  voltage u_a_filt1 : nesl_utility/PS-Simulink Converter  PhysicalDomain=network_engine_domain  SubClassName=ps_output  LeftPortType=input  RightPortType=output  PseudoPeriodic=off  Frequencies=[]  Unit=V  AffineConversion=off
      settings: SourceProductBaseCode=PW,SS
  voltage u_b_filt1 : nesl_utility/PS-Simulink Converter  PhysicalDomain=network_engine_domain  SubClassName=ps_output  LeftPortType=input  RightPortType=output  PseudoPeriodic=off  Frequencies=[]  Unit=V  AffineConversion=off
      settings: SourceProductBaseCode=PW,SS
  voltage u_c_filt1 : nesl_utility/PS-Simulink Converter  PhysicalDomain=network_engine_domain  SubClassName=ps_output  LeftPortType=input  RightPortType=output  PseudoPeriodic=off  Frequencies=[]  Unit=V  AffineConversion=off
      settings: SourceProductBaseCode=PW,SS
  HB1T : PMIOPort  Side=Left
  HB1B : PMIOPort  Port=2  Side=Left
  HB2T : PMIOPort  Port=3  Side=Left
  HB2B : PMIOPort  Port=4  Side=Left
  HB3T : PMIOPort  Port=5  Side=Left
  HB3B : PMIOPort  Port=6  Side=Left
  U_dc_+ : PMIOPort  Port=7  Side=Left
  U_dc_- : PMIOPort  Port=8  Side=Left
  u_1_ph : PMIOPort  Port=9  Side=Right
  u_2_ph : PMIOPort  Port=10  Side=Right
  u_3_ph : PMIOPort  Port=11  Side=Right
  i_1 : Outport  VectorParamsAs1DForOutWhenUnconnected=off
  i_2 : Outport  Port=2  VectorParamsAs1DForOutWhenUnconnected=off
  i_3 : Outport  Port=3  VectorParamsAs1DForOutWhenUnconnected=off
  i_dc : Outport  Port=4  VectorParamsAs1DForOutWhenUnconnected=off
  u_1_gnd : Outport  Port=5  VectorParamsAs1DForOutWhenUnconnected=off
  u_2_gnd : Outport  Port=6  VectorParamsAs1DForOutWhenUnconnected=off
  u_3_gnd : Outport  Port=7  VectorParamsAs1DForOutWhenUnconnected=off
  wires:
  PS-Simulink Converter/1 -> i_1/1
  PS-Simulink Converter1/1 -> i_2/1
  PS-Simulink Converter2/1 -> i_3/1
  PS-Simulink Converter12/1 -> i_dc/1
  12bit ADC1/1(y) -> Gain3/1
  voltage u_c_filt1/1 -> 12bit ADC2/1(u)
  Gain4/1 -> u_3_gnd/1
  12bit ADC2/1(y) -> Gain4/1
  12bit ADC/1(y) -> Gain2/1
  Gain2/1 -> u_1_gnd/1
  Gain3/1 -> u_2_gnd/1
  voltage u_b_filt1/1 -> 12bit ADC1/1(u)
  voltage u_a_filt1/1 -> 12bit ADC/1(u)
  PS-Simulink Converter6/1 -> u_dc/1
  volt_u1/1 -> To Workspace/1, Scope/1
  connections:
  MOSFET2/RConn2 -- Diode1/LConn1 -- i_2_ph/LConn1 -- Diode4/RConn1 -- MOSFET3/RConn1
  MOSFET/RConn1 -- Diode/RConn1 -- Diode2/RConn1 -- MOSFET4/RConn1 -- Diode1/RConn1 -- MOSFET2/RConn1 -- u_DC/LConn1 -- U_dc_+/RConn1
  MOSFET4/RConn2 -- Diode2/LConn1 -- i_3_ph/LConn1 -- Diode5/RConn1 -- MOSFET5/RConn1
  MOSFET2/LConn1 -- HB2T/RConn1
  MOSFET/LConn1 -- HB1T/RConn1
  MOSFET5/LConn1 -- HB3B/RConn1
  MOSFET1/LConn1 -- HB1B/RConn1
  MOSFET4/LConn1 -- HB3T/RConn1
  MOSFET3/LConn1 -- HB2B/RConn1
  i_1_ph/RConn2 -- 95,3kOhm/LConn1 -- Voltage Sensor/LConn1 -- u_1_ph/RConn1
  i_2_ph/RConn2 -- 95,3kOhm4/LConn1 -- u_2_ph/RConn1
  i_3_ph/RConn2 -- 95,3kOhm5/LConn1 -- u_3_ph/RConn1
  PS-Simulink Converter/LConn1 -- i_1_ph/RConn1
  PS-Simulink Converter1/LConn1 -- i_2_ph/RConn1
  PS-Simulink Converter2/LConn1 -- i_3_ph/RConn1
  PS-Simulink Converter12/LConn1 -- i_dc_ph/RConn1
  U_dc_-/RConn1 -- i_dc_ph/RConn2 -- u_DC/RConn2
  95,3kOhm5/RConn1 -- 0.1µF2/LConn1 -- u_c_filt/LConn1 -- 4,99kOhm2/LConn1
  0.1µF1/LConn1 -- u_b_filt/LConn1 -- 4,99kOhm1/LConn1 -- 95,3kOhm4/RConn1
  u_a_filt/LConn1 -- 0.1µF/LConn1 -- 4,99kOhm/LConn1 -- 95,3kOhm/RConn1
  voltage u_c_filt1/LConn1 -- u_c_filt/RConn1
  voltage u_a_filt1/LConn1 -- u_a_filt/RConn1
  voltage u_b_filt1/LConn1 -- u_b_filt/RConn1
  MOSFET5/RConn2 -- Diode5/LConn1 -- Voltage Sensor/RConn2 -- 0.1µF2/RConn1 -- 4,99kOhm2/RConn1 -- 4,99kOhm1/RConn1 -- 0.1µF1/RConn1 -- 4,99kOhm/RConn1 -- 0.1µF/RConn1 -- u_a_filt/RConn2 -- u_b_filt/RConn2 -- u_c_filt/RConn2 -- Diode4/LConn1 -- MOSFET3/RConn2 -- Diode3/LConn1 -- MOSFET1/RConn2 -- i_dc_ph/LConn1
  MOSFET/RConn2 -- i_1_ph/LConn1 -- Diode3/RConn1 -- MOSFET1/RConn1 -- Diode/LConn1
  u_DC/RConn1 -- PS-Simulink Converter6/LConn1
  volt_u1/LConn1 -- Voltage Sensor/RConn1

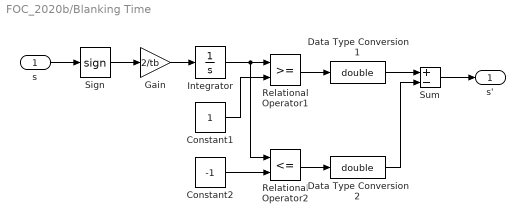
== system FOC_2020b/Blanking Time ==
  s : Inport
  Constant1 : Constant
  Constant2 : Constant  Value=-1
  Data Type Conversion1 : DataTypeConversion  OutDataTypeStr=double  SaturateOnIntegerOverflow=on  RndMeth=Zero
  Data Type Conversion2 : DataTypeConversion  OutDataTypeStr=double  SaturateOnIntegerOverflow=on  RndMeth=Zero
  Gain : Gain  Gain=2/tb  SaturateOnIntegerOverflow=on  OutDataTypeStr=Inherit: Same as input  ParamDataTypeStr=Inherit: Same as input
  Integrator : Integrator  LimitOutput=on  UpperSaturationLimit=1  LowerSaturationLimit=-1
  Relational Operator1 : RelationalOperator  RndMeth=Nearest  InputSameDT=on
  Relational Operator2 : RelationalOperator  Operator=<=  RndMeth=Nearest  InputSameDT=on
  Sign : Signum
  Sum : Sum  Inputs=+-  InputSameDT=on  SaturateOnIntegerOverflow=on  OutDataTypeStr=Inherit: Same as first input
  s' : Outport  VectorParamsAs1DForOutWhenUnconnected=off
  wires:
  Data Type Conversion2/1 -> Sum/2
  Relational Operator2/1 -> Data Type Conversion2/1
  Data Type Conversion1/1 -> Sum/1
  Relational Operator1/1 -> Data Type Conversion1/1
  Sum/1 -> s'/1
  Integrator/1 -> Relational Operator2/1, Relational Operator1/1
  Constant1/1 -> Relational Operator1/2
  Constant2/1 -> Relational Operator2/2
  Gain/1 -> Integrator/1
  Sign/1 -> Gain/1
  s/1 -> Sign/1

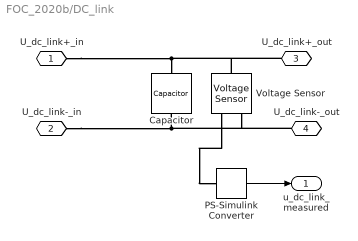
== system FOC_2020b/DC_link ==
  Capacitor : fl_lib/Electrical/Electrical Elements/Capacitor  c=C_dc_link uF  r=1e-6 Ohm  g=0 1/Ohm  i_specify=off  i_priority=None  i=0 A  i_nominal_specify=off  i_nominal_unit=A  i_nominal_value=1  v_specify=off  v_priority=None  v=0 V  v_nominal_specify=off  v_nominal_unit=V  v_nominal_value=1  vc_specify=off  vc_priority=High  vc=0 V  vc_nominal_specify=off  vc_nominal_unit=V  vc_nominal_value=1
  PS-Simulink Converter : nesl_utility/PS-Simulink Converter  PhysicalDomain=network_engine_domain  SubClassName=ps_output  LeftPortType=input  RightPortType=output  PseudoPeriodic=off  Frequencies=[]  Unit=1  AffineConversion=off
      settings: SourceProductBaseCode=PW,SS
  Voltage Sensor : fl_lib/Electrical/Electrical Sensors/Voltage Sensor
  U_dc_link+_in : PMIOPort  Side=Left
  U_dc_link-_in : PMIOPort  Port=2  Side=Left
  U_dc_link+_out : PMIOPort  Port=3  Side=Right
  U_dc_link-_out : PMIOPort  Port=4  Side=Right
  u_dc_link_measured : Outport  VectorParamsAs1DForOutWhenUnconnected=off
  wires:
  PS-Simulink Converter/1 -> u_dc_link_measured/1
  connections:
  U_dc_link+_in/RConn1 -- Voltage Sensor/LConn1 -- U_dc_link+_out/RConn1 -- Capacitor/LConn1
  U_dc_link-_in/RConn1 -- Voltage Sensor/RConn2 -- U_dc_link-_out/RConn1 -- Capacitor/RConn1
  Voltage Sensor/RConn1 -- PS-Simulink Converter/LConn1
